simulink model "Question_6_a"  (R2014a)
settings: Solver=ode45  StartTime=0.0  StopTime=10.0  RelTol=1e-3
settings Model: Creator=Shiyu  LastModifiedBy=Shiyu

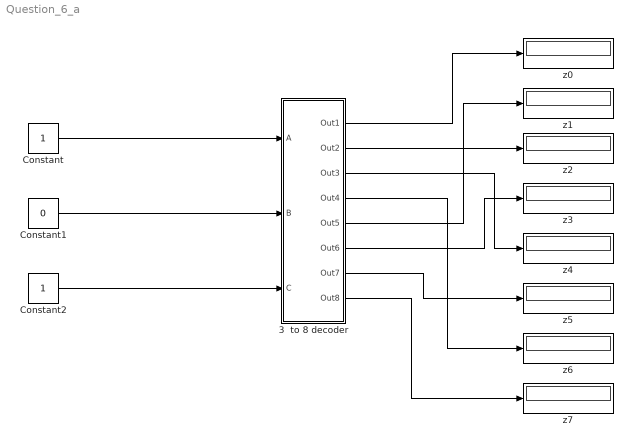
== system Question_6_a ==
  "3  to 8 decoder " : Subsystem
  Constant : Constant  OutDataTypeStr=boolean
  Constant1 : Constant  Value=0  OutDataTypeStr=boolean
  Constant2 : Constant  OutDataTypeStr=boolean
  z{0..7} (8 alike) : Display
  wires:
  Constant/1 -> "3  to 8 decoder "/1(A)
  Constant1/1 -> "3  to 8 decoder "/2(B)
  Constant2/1 -> "3  to 8 decoder "/3(C)
  "3  to 8 decoder "/1(Out1) -> z0/1
  "3  to 8 decoder "/2(Out2) -> z2/1
  "3  to 8 decoder "/3(Out3) -> z4/1
  "3  to 8 decoder "/4(Out4) -> z6/1
  "3  to 8 decoder "/5(Out5) -> z1/1
  "3  to 8 decoder "/6(Out6) -> z3/1
  "3  to 8 decoder "/7(Out7) -> z5/1
  "3  to 8 decoder "/8(Out8) -> z7/1

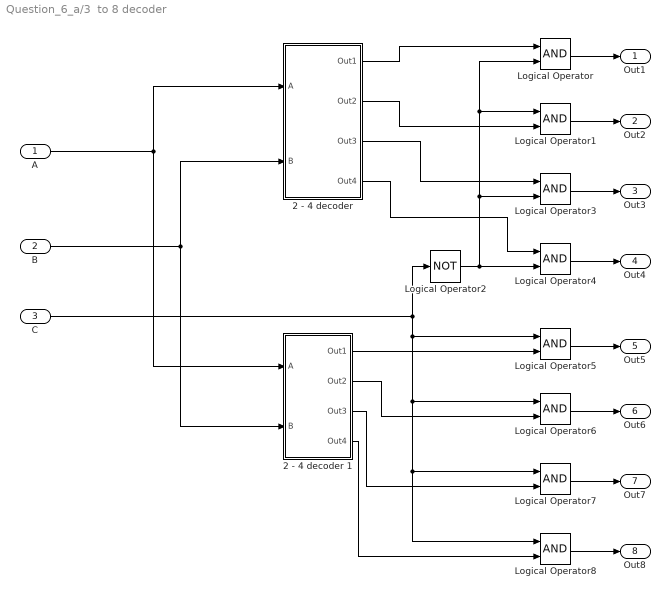
== system Question_6_a/3  to 8 decoder  ==
  A : Inport  OutDataTypeStr=boolean  SampleTime=1
  B : Inport  Port=2  OutDataTypeStr=boolean  SampleTime=1
  C : Inport  Port=3  OutDataTypeStr=boolean  SampleTime=1
  "2 - 4 decoder " : Subsystem
  2 - 4 decoder 1 : Subsystem
  Logical Operator{,1,3..8} (8 alike) : Logic  AllPortsSameDT=off  OutDataTypeStr=boolean
  Logical Operator2 : Logic  Operator=NOT  AllPortsSameDT=off  OutDataTypeStr=boolean
  Out1 : Outport
  Out2 : Outport  Port=2
  Out3 : Outport  Port=3
  Out4 : Outport  Port=4
  Out5 : Outport  Port=5
  Out6 : Outport  Port=6
  Out7 : Outport  Port=7
  Out8 : Outport  Port=8
  wires:
  Logical Operator3/1 -> Out3/1
  B/1 -> 2 - 4 decoder 1/2(B), "2 - 4 decoder "/2(B)
  A/1 -> 2 - 4 decoder 1/1(A), "2 - 4 decoder "/1(A)
  "2 - 4 decoder "/1(Out1) -> Logical Operator/1
  "2 - 4 decoder "/2(Out2) -> Logical Operator1/2
  Logical Operator7/1 -> Out7/1
  2 - 4 decoder 1/4(Out4) -> Logical Operator8/2
  "2 - 4 decoder "/4(Out4) -> Logical Operator4/1
  Logical Operator4/1 -> Out4/1
  Logical Operator1/1 -> Out2/1
  "2 - 4 decoder "/3(Out3) -> Logical Operator3/1
  Logical Operator/1 -> Out1/1
  2 - 4 decoder 1/3(Out3) -> Logical Operator7/2
  C/1 -> Logical Operator8/1, Logical Operator7/1, Logical Operator6/1, Logical Operator5/1, Logical Operator2/1
  Logical Operator8/1 -> Out8/1
  2 - 4 decoder 1/1(Out1) -> Logical Operator5/2
  Logical Operator6/1 -> Out6/1
  Logical Operator2/1 -> Logical Operator4/2, Logical Operator/2, Logical Operator1/1, Logical Operator3/2
  2 - 4 decoder 1/2(Out2) -> Logical Operator6/2
  Logical Operator5/1 -> Out5/1

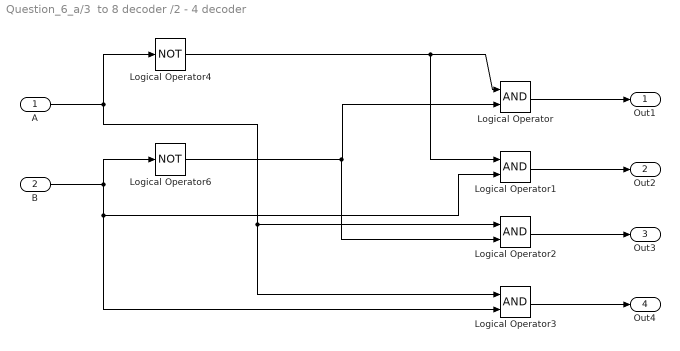
== system Question_6_a/3  to 8 decoder /2 - 4 decoder  ==
  A : Inport
  B : Inport  Port=2
  Logical Operator{,1..3} (4 alike) : Logic  AllPortsSameDT=off  OutDataTypeStr=boolean
  Logical Operator4 : Logic  Operator=NOT  AllPortsSameDT=off  OutDataTypeStr=boolean
  Logical Operator6 : Logic  Operator=NOT  AllPortsSameDT=off  OutDataTypeStr=boolean
  Out1 : Outport
  Out2 : Outport  Port=2
  Out3 : Outport  Port=3
  Out4 : Outport  Port=4
  wires:
  Logical Operator6/1 -> Logical Operator2/2, Logical Operator/2
  A/1 -> Logical Operator3/1, Logical Operator2/1, Logical Operator4/1
  Logical Operator3/1 -> Out4/1
  Logical Operator/1 -> Out1/1
  B/1 -> Logical Operator6/1, Logical Operator3/2, Logical Operator1/2
  Logical Operator2/1 -> Out3/1
  Logical Operator4/1 -> Logical Operator1/1, Logical Operator/1
  Logical Operator1/1 -> Out2/1

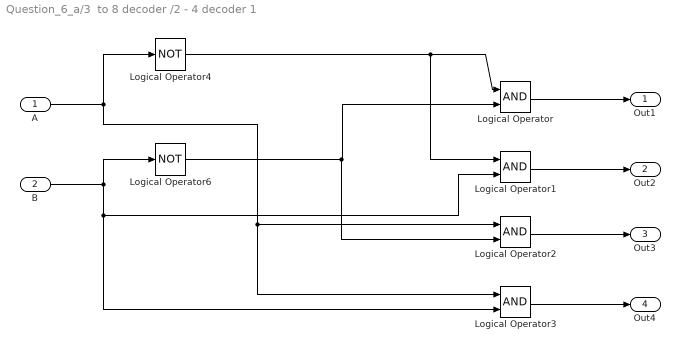
== system Question_6_a/3  to 8 decoder /2 - 4 decoder 1 ==
  A : Inport
  B : Inport  Port=2
  Logical Operator{,1..3} (4 alike) : Logic  AllPortsSameDT=off  OutDataTypeStr=boolean
  Logical Operator4 : Logic  Operator=NOT  AllPortsSameDT=off  OutDataTypeStr=boolean
  Logical Operator6 : Logic  Operator=NOT  AllPortsSameDT=off  OutDataTypeStr=boolean
  Out1 : Outport
  Out2 : Outport  Port=2
  Out3 : Outport  Port=3
  Out4 : Outport  Port=4
  wires:
  Logical Operator6/1 -> Logical Operator2/2, Logical Operator/2
  A/1 -> Logical Operator3/1, Logical Operator2/1, Logical Operator4/1
  Logical Operator3/1 -> Out4/1
  Logical Operator/1 -> Out1/1
  B/1 -> Logical Operator6/1, Logical Operator3/2, Logical Operator1/2
  Logical Operator2/1 -> Out3/1
  Logical Operator4/1 -> Logical Operator1/1, Logical Operator/1
  Logical Operator1/1 -> Out2/1
